simulink model "lab2_4"  (Simulink 7.9)
settings: Solver=ode45  StartTime=0.0  StopTime=0.3  RelTol=1e-3
libraries: simulink x1
settings Model: Creator=Aquirel  LastModifiedBy=Aquirel

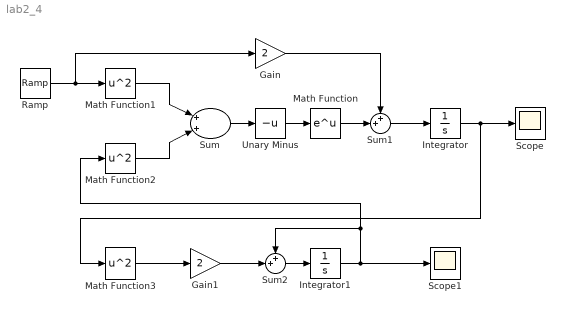
== system lab2_4 ==
  Gain : Gain  Gain=2
  Gain1 : Gain  Gain=2
  Integrator : Integrator  InitialCondition=0.5
  Integrator1 : Integrator  InitialCondition=1
  Math Function : Math  SaturateOnIntegerOverflow=on
  Math Function1 : Math  Operator=square  SaturateOnIntegerOverflow=on
  Math Function2 : Math  Operator=square  SaturateOnIntegerOverflow=on
  Math Function3 : Math  Operator=square  SaturateOnIntegerOverflow=on
  Ramp : simulink/Sources/Ramp  slope=1  start=0  X0=0
  Scope : Scope
      settings: YMin=0  YMax=1.7
  Scope1 : Scope
      settings: YMin=0  YMax=1.7
  Sum : Sum  Inputs=|++|
  Sum1 : Sum  Inputs=++|
  Sum2 : Sum  Inputs=++|
  Unary Minus : UnaryMinus
  wires:
  Unary Minus/1 -> Math Function/1
  Sum/1 -> Unary Minus/1
  Math Function1/1 -> Sum/1
  Math Function2/1 -> Sum/2
  Ramp/1 -> Math Function1/1, Gain/1
  Math Function/1 -> Sum1/2
  Gain/1 -> Sum1/1
  Sum1/1 -> Integrator/1
  Math Function3/1 -> Gain1/1
  Gain1/1 -> Sum2/2
  Sum2/1 -> Integrator1/1
  Integrator1/1 -> Scope1/1, Sum2/1, Math Function2/1
  Integrator/1 -> Math Function3/1, Scope/1
